simulink model "Hele_modellen_24_05_kl_20"  (R2022b)
settings: Solver=ode23t  StartTime=0.0  StopTime=3000  RelTol=1e-3
values from neighbouring files (symbols this model uses):
  A_stack_surface = 0.8*0.97*2+0.8*1.5*2+0.97*1.5*2    (= 6.862)    [Alle_konstanter_24_5_kl_20.m]
  c_p_stack = 870    [Alle_konstanter_24_5_kl_20.m]
  c_p_w = nyeretabelTcp.VarName2(1:250)    [Alle_konstanter_24_5_kl_20.m]
  cell_area = 5600    [Alle_konstanter_24_5_kl_20.m]
  ctc_an = 2    [Alle_konstanter_24_5_kl_20.m]
  ctc_ca = 2    [Alle_konstanter_24_5_kl_20.m]
  F = 96485.3321233100184    (= 96485.3321233)    [Alle_konstanter_24_5_kl_20.m]
  h_conv = 7.5    [Alle_konstanter_24_5_kl_20.m]
  i_0_an = 2*10^(-7)    (= 2e-07)    [Alle_konstanter_24_5_kl_20.m]
  i_0_ca = 2*10^(-3)    (= 0.002)    [Alle_konstanter_24_5_kl_20.m]
  idensdata = [0.746899 0.747476 0.748293 0.748876 0.749145 0.749908 0.750254 0.75072 0.751353 0.751779 0.752202 0.752682 ... (7200 elements, 90x80)]    [idensdata.mat]    (also in park_power.mat)
  lambda_m = 21    [Alle_konstanter_24_5_kl_20.m]
  M_H2 = 0.002016    [Alle_konstanter_24_5_kl_20.m]
  M_O2 = 0.031999    [Alle_konstanter_24_5_kl_20.m]
  m_stack = 2300    [Alle_konstanter_24_5_kl_20.m]
  N_cell = 36    [Alle_konstanter_24_5_kl_20.m]
  nr_of_stacks = 7    [Alle_konstanter_24_5_kl_20.m]
  P_lookup = 2:0.1:9.9    [Alle_konstanter_24_5_kl_20.m]
  R = 8.314    [Alle_konstanter_24_5_kl_20.m]
  T = transpose(1:250)    [Alle_konstanter_24_5_kl_20.m]
  T_amb = 20    [Alle_konstanter_24_5_kl_20.m]
  T_lookup = 283.15:1:372.15    [Alle_konstanter_24_5_kl_20.m]
  t_me = 175*10^(-4)    (= 0.0175)    [Alle_konstanter_24_5_kl_20.m]
  U_th = 1.473    [Alle_konstanter_24_5_kl_20.m]
undefined symbols (not defined in the file or in its folder): DiscIntNeverNeededParam
libraries: fl_lib x17, nesl_utility x10, ee_lib x2, SimscapeFluids_lib x1, simulink x1, dspsrcs4 x1
settings Model: Creator=drjon  LastModifiedBy=IrisM

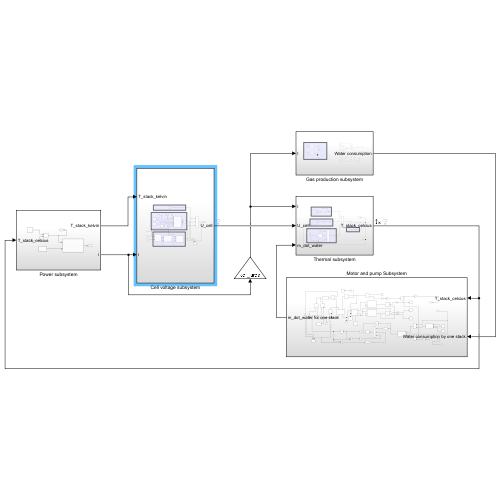
[thumbnail: Simulink's stored preview of the top-level diagram]
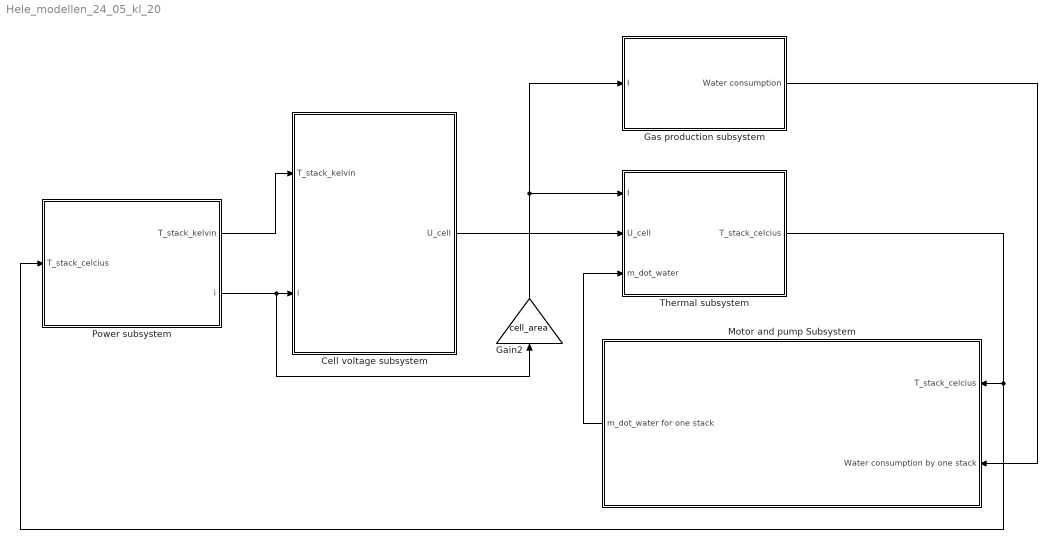
== system Hele_modellen_24_05_kl_20 ==
  Cell voltage subsystem : Subsystem
  Gain2 : Gain  Gain=cell_area
  Gas production subsystem : Subsystem
  Motor and pump Subsystem : Subsystem
  Power subsystem : Subsystem
  Thermal subsystem : Subsystem
  wires:
  Thermal subsystem/1(T_stack_celcius) -> Power subsystem/1(T_stack_celcius), Motor and pump Subsystem/1(T_stack_celcius)
  Cell voltage subsystem/1(U_cell) -> Thermal subsystem/2(U_cell)
  Gain2/1 -> Gas production subsystem/1(I), Thermal subsystem/1(I)
  Gas production subsystem/1(Water consumption) -> Motor and pump Subsystem/2(Water consumption by one stack)
  Motor and pump Subsystem/1(m_dot_water for one stack) -> Thermal subsystem/3(m_dot_water)
  Power subsystem/2(i) -> Cell voltage subsystem/2(i), Gain2/1
  Power subsystem/1(T_stack_kelvin) -> Cell voltage subsystem/1(T_stack_kelvin)

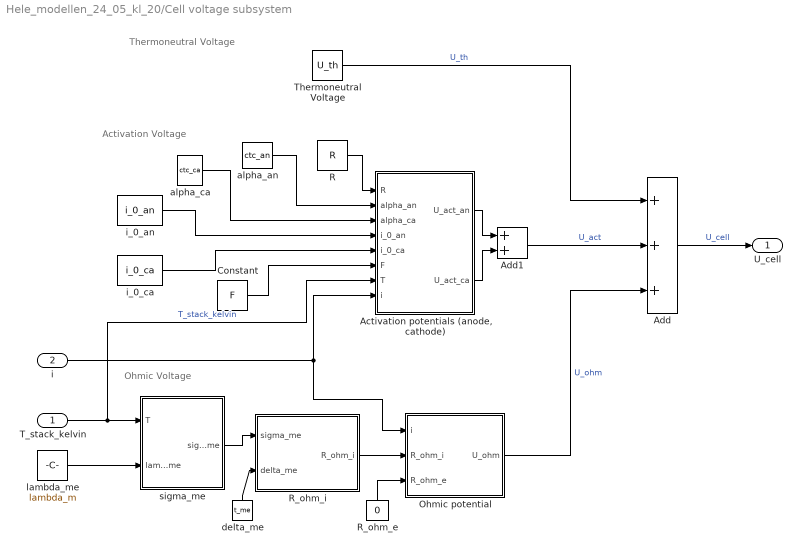
== system Hele_modellen_24_05_kl_20/Cell voltage subsystem ==
  note: Ohmic Voltage
  note: Activation Voltage
  note: Thermoneutral Voltage
  T_stack_kelvin : Inport
  i : Inport  Port=2
  "Activation potentials (anode, cathode)" : MATLAB Function  TreatAsAtomicUnit=on
  Add : Sum  Inputs=+++
  Add1 : Sum
  Constant : Constant  Value=F
  Ohmic potential : MATLAB Function  TreatAsAtomicUnit=on
  R : Constant  Value=R
  R_ohm_e : Constant  Value=0
  R_ohm_i : MATLAB Function  TreatAsAtomicUnit=on
  Thermoneutral Voltage : Constant  Value=U_th
  alpha_an : Constant  Value=ctc_an
  alpha_ca : Constant  Value=ctc_ca
  delta_me : Constant  Value=t_me
  i_0_an : Constant  Value=i_0_an
  i_0_ca : Constant  Value=i_0_ca
  lambda_me : Constant  Value=lambda_m
  sigma_me : MATLAB Function  TreatAsAtomicUnit=on
  U_cell : Outport
  wires:
  lambda_me/1 -> sigma_me/2(lambda_me)
  T_stack_kelvin/1 -> "Activation potentials (anode, cathode)"/7(T), sigma_me/1(T)  "T_stack_kelvin"
  i_0_an/1 -> "Activation potentials (anode, cathode)"/4(i_0_an)
  R/1 -> "Activation potentials (anode, cathode)"/1(R)
  i_0_ca/1 -> "Activation potentials (anode, cathode)"/5(i_0_ca)
  R_ohm_i/1(R_ohm_i) -> Ohmic potential/2(R_ohm_i)
  Add/1 -> U_cell/1  "U_cell"
  Add1/1 -> Add/2  "U_act"
  alpha_an/1 -> "Activation potentials (anode, cathode)"/2(alpha_an)
  delta_me/1 -> R_ohm_i/2(delta_me)
  Ohmic potential/1(U_ohm) -> Add/3  "U_ohm"
  sigma_me/1(sigma_me) -> R_ohm_i/1(sigma_me)
  alpha_ca/1 -> "Activation potentials (anode, cathode)"/3(alpha_ca)
  R_ohm_e/1 -> Ohmic potential/3(R_ohm_e)
  Constant/1 -> "Activation potentials (anode, cathode)"/6(F)
  Thermoneutral Voltage/1 -> Add/1  "U_th"
  "Activation potentials (anode, cathode)"/1(U_act_an) -> Add1/1
  "Activation potentials (anode, cathode)"/2(U_act_ca) -> Add1/2
  i/1 -> "Activation potentials (anode, cathode)"/8(i), Ohmic potential/1(i)

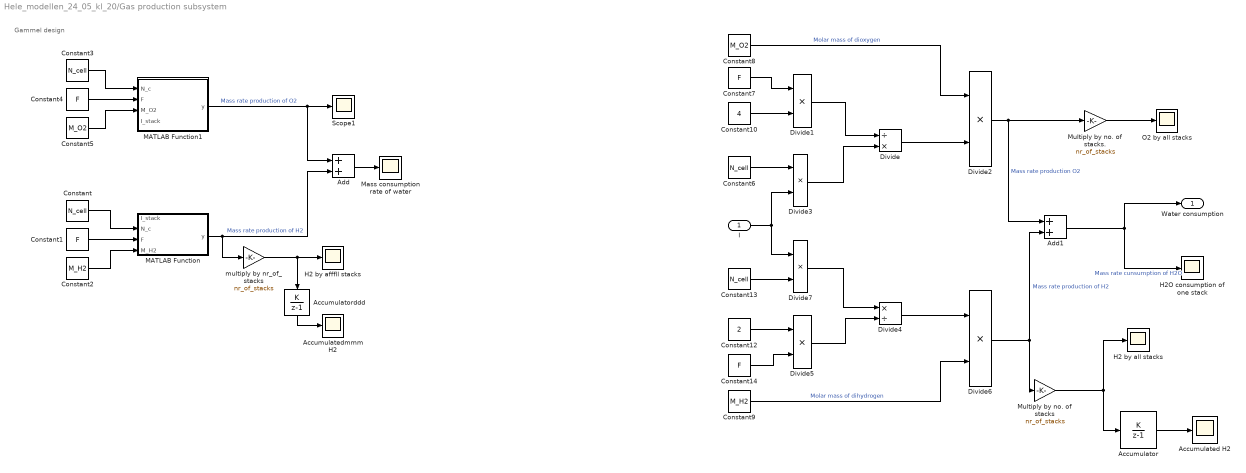
== system Hele_modellen_24_05_kl_20/Gas production subsystem ==
  note: Gammel design
  I : Inport
  Accumulated H2 : Scope
  Accumulatedmmm H2 : Scope
  Accumulator : DiscreteIntegrator  IntegratorMethod=Accumulation: Forward Euler  SampleTime=-1  ICPrevOutput=DiscIntNeverNeededParam  ICPrevScaledInput=DiscIntNeverNeededParam
  Accumulatorddd : DiscreteIntegrator  IntegratorMethod=Accumulation: Forward Euler  SampleTime=-1  ICPrevOutput=DiscIntNeverNeededParam  ICPrevScaledInput=DiscIntNeverNeededParam
  Add : Sum
  Add1 : Sum
  Constant{,3,6,13} (4 alike) : Constant  Value=N_cell
  Constant{1,4,7,14} (4 alike) : Constant  Value=F
  Constant10 : Constant  Value=4
  Constant12 : Constant  Value=2
  Constant2 : Constant  Value=M_H2
  Constant5 : Constant  Value=M_O2
  Constant8 : Constant  Value=M_O2
  Constant9 : Constant  Value=M_H2
  Divide : Product  Inputs=/*
  Divide{1..3,5..7} (6 alike) : Product  Inputs=**
  Divide4 : Product  Inputs=*/
  H2 by afffll stacks : Scope
  H2 by all stacks : Scope
  H2O consumption of one stack : Scope
  MATLAB Function : MATLAB Function  TreatAsAtomicUnit=on
  MATLAB Function1 : MATLAB Function  TreatAsAtomicUnit=on
  Mass consumption rate of water : Scope
  Multiply by no. of stacks : Gain  Gain=nr_of_stacks
  Multiply by no. of stacks. : Gain  Gain=nr_of_stacks
  O2 by all stacks : Scope
  Scope1 : Scope
  multiply by nr_of_stacks : Gain  Gain=nr_of_stacks
  Water consumption : Outport
  wires:
  MATLAB Function1/1(y) -> Add/1, Scope1/1  "Mass rate production of O2"
  Constant/1 -> MATLAB Function/2(N_c)
  Constant1/1 -> MATLAB Function/3(F)
  Add/1 -> Mass consumption rate of water/1
  Constant2/1 -> MATLAB Function/4(M_H2)
  Constant4/1 -> MATLAB Function1/2(F)
  MATLAB Function/1(y) -> Add/2, multiply by nr_of_stacks/1  "Mass rate production of H2"
  Constant5/1 -> MATLAB Function1/3(M_O2)
  Constant3/1 -> MATLAB Function1/1(N_c)
  multiply by nr_of_stacks/1 -> H2 by afffll stacks/1, Accumulatorddd/1
  Accumulatorddd/1 -> Accumulatedmmm H2/1
  Constant12/1 -> Divide5/1
  Constant7/1 -> Divide1/1
  Divide7/1 -> Divide4/1
  Divide3/1 -> Divide/2
  Multiply by no. of stacks/1 -> H2 by all stacks/1, Accumulator/1
  Divide4/1 -> Divide6/1
  Constant9/1 -> Divide6/2  "Molar mass of dihydrogen"
  Divide5/1 -> Divide4/2
  Constant14/1 -> Divide5/2
  Divide1/1 -> Divide/1
  Constant13/1 -> Divide7/2
  Constant8/1 -> Divide2/1  "Molar mass of dioxygen"
  Add1/1 -> Water consumption/1, H2O consumption of one stack/1  "Mass rate cunsumption of H2O"
  Constant10/1 -> Divide1/2
  Divide6/1 -> Add1/2, Multiply by no. of stacks/1  "Mass rate production of H2"
  Divide/1 -> Divide2/2
  Constant6/1 -> Divide3/1
  Divide2/1 -> Multiply by no. of stacks./1, Add1/1  "Mass rate production O2"
  Accumulator/1 -> Accumulated H2/1
  I/1 -> Divide7/1, Divide3/2
  Multiply by no. of stacks./1 -> O2 by all stacks/1

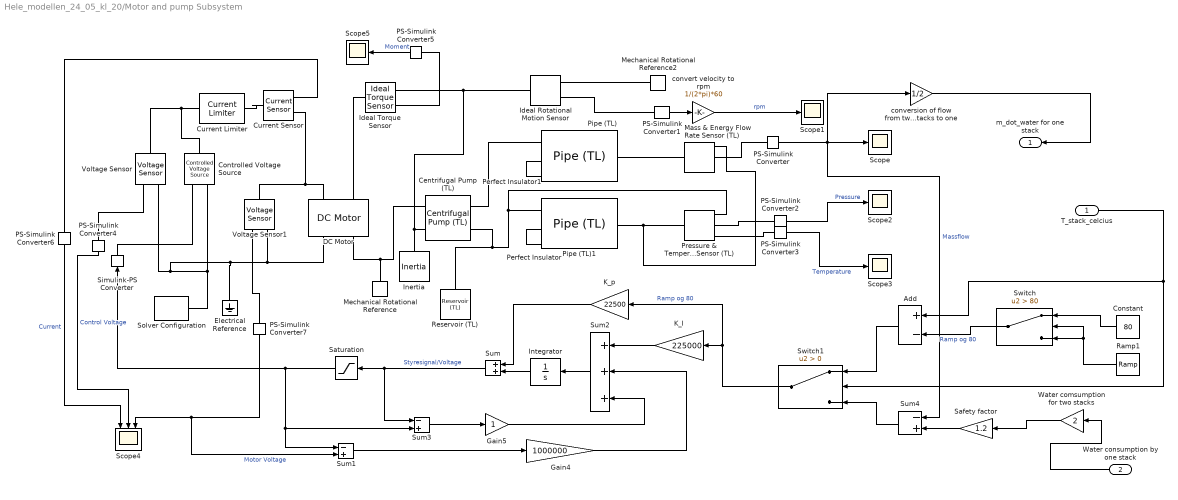
== system Hele_modellen_24_05_kl_20/Motor and pump Subsystem ==
  T_stack_celcius : Inport
  Water consumption by one stack : Inport  Port=2
  Add : Sum  Inputs=+-
  Centrifugal Pump (TL) : SimscapeFluids_lib/Thermal Liquid/Pumps & Motors/Centrifugal Pump (TL)  pump_parameterization=fluids.thermal_liquid.pumps_motors.enum.CentrifugalPumpParameterization.Nominal  capacity_ref_nominal=290 lpm  head_ref_nominal=40 m  power_ref_nominal=0.85 kW  head_ref_max=60 m  capacity_ref_max=300 lpm  omega_ref_analytic=1150 rpm  flow_rate_1D_TLU=[16.67, 30, 40, 53.33, 66.67, 83.33] lpm  head_1D_TLU=[50, 47.5, 45, 40, 35, 25] m  power_1D_TLU=[.6, .75, .85, .93, .98, .99] kW  omega_ref_1D=3500 rpm  rho_ref_1D=998.21 kg/m^3  flow_rate_2D_TLU=[16.67, 23.33, 30, 40, 53.33, 60] lpm  omega_2D_TLU=[2450, 2800, 3150, 3500] rpm  head_2D_TLU=[25, 32.7, 42.5, 50; 24, 31.7, 41, 49; 22.7, 30.5, 39, 47.5; 20, 28, 36, 45; 15.7, 24, 32, 40; 12.5, 21, 29.5, 37.5] m  power_2D_TLU=[.28, .38, .5, .6; .31, .41, .55, .68; .33, .44, .6, .75; .36, .48, .65, .83; .38, .53, .72, .93; .39, .55, .75, .97] kW  rho_ref_2D=998.21 kg/m^3  diameter_ratio=1  mech_orientation=fluids.thermal_liquid.pumps_motors.enum.CentrifugalPumpMechOrientation.Positive  area=0.01 m^2
      settings: InternalSimscapePortConfiguration="{\"Bottom\":[],\"Left\":[{\"id\":\"A\",\"label\":\"A\",\"type\":\"foundation.thermal_liquid.thermal_liquid\"},{\"id\":\"B\",\"label\":\"B\",\"type\":\"foundation.thermal_liquid.thermal_liquid\"}],\"Right\":[{\"id\":\"R\",\"label\":\"R\",\"type\":\"foundation.mechanical.rotational.rotational\"},{\"id\":\"C\",\"label\":\"C\",\"type\":\"foundation.mechanical.rotational.rotational\"}],\"Top\":[]}"
  Constant : Constant  Value=80
  Controlled Voltage Source : fl_lib/Electrical/Electrical Sources/Controlled Voltage Source
  Current Limiter : ee_lib/Semiconductors & Converters/Current Limiter  iLim=4.5 A  vLim=0.1 V  gLim=1e-9 1/Ohm  thermal_mass=100 J/K  initial_temperature=298.15 K
      settings: InternalSimscapePortConfiguration="{\"Bottom\":[],\"Left\":[{\"id\":\"p\",\"label\":\"+\",\"type\":\"foundation.electrical.electrical\"}],\"Right\":[{\"id\":\"n\",\"label\":\"-\",\"type\":\"foundation.electrical.electrical\"}],\"Top\":[]}"
  Current Sensor : fl_lib/Electrical/Electrical Sensors/Current Sensor
  DC Motor : ee_lib/Electromechanical/Brushed Motors/DC Motor  field_option=ee.enum.field_option.pm  Rf=100 Ohm  Lf=1 H  Laf=0.15 H  If0=0 A  parameterization=ee.enum.dcparam_option.circuit_param  Ra=3.9 Ohm  La=14e-3 H  emf_or_torque=ee.enum.emf_or_torque.kv  Kv=1.2 V/(rad/s)  Ki=6.876e-4 N*m/A  T_stall=0.24e-3 N*m  w_max=19100 rpm  w_rated=15000 rpm  P_rated=0.08 W  V_rated=1.5 V  lam_param=ee.enum.lam_param.damping  i_noload=0 A  V_i_noload=1.5 V  J=0.00088 kg*m^2  lam=0 N*m*s/rad  speed0=0 rpm  enable_fault_armature=simscape.enum.onoff.off  rev_faulted=1 / 3  G_faulted_armature=1e-5 S  fault_trigger_armature=ee.enum.faults.faultTrigger.temporal  t_fault_armature=1 s  max_permissible_current_armature=inf A  t_fail_on_current_armature=1 s  enable_fault_field=simscape.enum.onoff.off  G_faulted_field=1e-5 S  fault_trigger_field=ee.enum.faults.faultTrigger.temporal  t_fault_field=1 s  max_permissible_current_field=inf A  t_fail_on_current_field=1 s  fault_action=simscape.enum.assert.action.none  alpha=3.93e-3 1/K  Tmeas=25 degC  thermal_mass=100 J/K  initial_temperature=25 degC
  Electrical Reference : fl_lib/Electrical/Electrical Elements/Electrical Reference
  Gain4 : Gain  Gain=1000000
  Gain5 : Gain
  Ideal Rotational Motion Sensor : fl_lib/Mechanical/Mechanical Sensors/Ideal Rotational Motion Sensor  reference=foundation.enum.MeasurementReference.difference  acceleration_port=false  velocity_port=true  position_port=false  wrap_angle=false  offset=0 rad
      settings: InternalSimscapePortConfiguration="{\"Bottom\":[],\"Left\":[{\"id\":\"R\",\"label\":\"R\",\"type\":\"foundation.mechanical.rotational.rotational\"}],\"Right\":[{\"id\":\"C\",\"label\":\"C\",\"type\":\"foundation.mechanical.rotational.rotational\"},{\"id\":\"W\",\"label\":\"W\",\"type\":\"output\"}],\"Top\":[]}"
  Ideal Torque Sensor : fl_lib/Mechanical/Mechanical Sensors/Ideal Torque Sensor
  Inertia : fl_lib/Mechanical/Rotational Elements/Inertia  inertia=0.000176 kg*m^2  num_ports=foundation.enum.numPorts2.one  w_specify=off  w_priority=High  w=0 rad/s  w_nominal_specify=off  w_nominal_unit=rad/s  w_nominal_value=1  t_specify=off  t_priority=None  t=0 N*m  t_nominal_specify=off  t_nominal_unit=N*m  t_nominal_value=1
  Integrator : Integrator
  K_I : Gain  Gain=225000
  K_p : Gain  Gain=22500
  Mass & Energy Flow Rate Sensor (TL) : fl_lib/Thermal Liquid/Sensors/Mass & Energy Flow Rate Sensor (TL)
      settings: InternalSimscapePortConfiguration="{\"Bottom\":[],\"Left\":[{\"id\":\"A\",\"label\":\"A\",\"type\":\"foundation.thermal_liquid.thermal_liquid\"}],\"Right\":[{\"id\":\"B\",\"label\":\"B\",\"type\":\"foundation.thermal_liquid.thermal_liquid\"},{\"id\":\"M\",\"label\":\"M\",\"type\":\"output\"},{\"id\":\"PHI\",\"label\":\"Phi\",\"type\":\"output\"}],\"Top\":[]}"
  Mechanical Rotational Reference : fl_lib/Mechanical/Rotational Elements/Mechanical Rotational Reference
  Mechanical Rotational Reference2 : fl_lib/Mechanical/Rotational Elements/Mechanical Rotational Reference
  PS-Simulink Converter{,1..7} (8 alike) : nesl_utility/PS-Simulink Converter  PhysicalDomain=network_engine_domain  SubClassName=ps_output  LeftPortType=input  RightPortType=output  PseudoPeriodic=off  Frequencies=[]  VectorFormat=inherit  Unit=inherit  AffineConversion=off
  Perfect Insulator : fl_lib/Thermal/Thermal Elements/Perfect Insulator  T_specify=off  T_priority=None  T=293.15 K  T_nominal_specify=off  T_nominal_unit=K  T_nominal_value=1
  Perfect Insulator1 : fl_lib/Thermal/Thermal Elements/Perfect Insulator  T_specify=off  T_priority=None  T=293.15 K  T_nominal_specify=off  T_nominal_unit=K  T_nominal_value=1
  Pipe (TL) : fl_lib/Thermal Liquid/Elements/Pipe (TL)  length=5 m  area=0.01 m^2  Dh=0.1128 m  length_add=1 m  roughness=15e-6 m  Re_lam=2000  Re_tur=4000  shape_factor=64  Nu_lam=3.66  dynamic_compressibility=simscape.enum.onoff.on  inertia=simscape.enum.onoff.off  p0=3.5 MPa  T0=293.15 K  mdot0=0 kg/s
  Pipe (TL)1 : fl_lib/Thermal Liquid/Elements/Pipe (TL)  length=5 m  area=0.01 m^2  Dh=0.1128 m  length_add=1 m  roughness=15e-6 m  Re_lam=2000  Re_tur=4000  shape_factor=64  Nu_lam=3.66  dynamic_compressibility=simscape.enum.onoff.on  inertia=simscape.enum.onoff.off  p0=3.5 MPa  T0=293.15 K  mdot0=0 kg/s
  Pressure & Temperature Sensor (TL) : fl_lib/Thermal Liquid/Sensors/Pressure & Temperature Sensor (TL)
      settings: InternalSimscapePortConfiguration="{\"Bottom\":[],\"Left\":[{\"id\":\"A\",\"label\":\"A\",\"type\":\"foundation.thermal_liquid.thermal_liquid\"}],\"Right\":[{\"id\":\"B\",\"label\":\"B\",\"type\":\"foundation.thermal_liquid.thermal_liquid\"},{\"id\":\"P\",\"label\":\"P\",\"type\":\"output\"},{\"id\":\"T\",\"label\":\"T\",\"type\":\"output\"}],\"Top\":[]}"
  Ramp1 : simulink/Sources/Ramp  slope=0.05  start=0  InitialOutput=20
  Reservoir (TL) : fl_lib/Thermal Liquid/Elements/Reservoir (TL)  pressure_spec=foundation.enum.pressure_spec.specified  reservoir_pressure=3.5 MPa  reservoir_temperature=293.15 K  area=0.01 m^2
  Safety factor : Gain  Gain=1.2
  Saturation : Saturate  UpperLimit=300  LowerLimit=0
  Scope{,1..3,5} (5 alike) : Scope
  Scope4 : Scope  NumInputPorts=3
  Simulink-PS Converter : nesl_utility/Simulink-PS Converter  PhysicalDomain=network_engine_domain  SubClassName=ps_input  LeftPortType=input  RightPortType=output  PseudoPeriodic=off  Frequencies=[]  NoiseDistribution=none  NoiseParameters=[]  Unit=1  AffineConversion=off  FilteringAndDerivatives=provide  SimscapeFilterOrder=1  InputFilterTimeConstant=0.001  UdotUserProvided=0
  Solver Configuration : nesl_utility/Solver Configuration  PhysicalDomain=network_engine_domain  SubClassName=solver  LeftPortType=input  RightPortType=generic  Tones=[]  Harmonics=[]  SimulateNoise=off  Profile=off  UseLocalSampling=off  EnableSwitchedLinearOptims=on  FrequencyDomain=off  UseCCode=off  RelTol=0.001  AbsTol=0.001  MinStep=1e-09  ToWorkspace=off  RevertToSquareIcSolve=off  NumHomotopyIterations=100  PhasorMode=off  PhasorModeNumHarmonics=1  ConsistencySolver=NEWTON_XTOL_AFTER_FTOL  IndexReductionMethod=DerivativeReplacement  DoDC=off  ResidualTolerance=1e-09  ConsistencyTolSource=GLOBAL  ConsistencyAbsTol=0.001  ConsistencyRelTol=0.001  ConsistencyTolFactor=0.001  UseLocalSolver=off  LocalSolverChoice=NE_BACKWARD_EULER_ADVANCER  ResolveIndetEquations=on  FunctionEvalNumThread=1  LocalSolverSampleTime=0.001  DoFixedCost=off  MaxNonlinIter=3  MaxModeIter=2  ComputeImpulses=off  ImpulseIterations=2  LinearAlgebra=auto  LinearAlgebraNumThread=0  EquationFormulation=NE_TIME_EF  DelaysMemoryBudget=1024  AutomaticFiltering=on  FilteringTimeConstant=0.001  PartitionStorageMethod=AS_NEEDED  PartitionMemoryBudget=1024  PartitionMethod=ROBUST
  Sum : Sum
  Sum1 : Sum  Inputs=-+
  Sum2 : Sum  Inputs=+++
  Sum3 : Sum  Inputs=-+
  Sum4 : Sum  Inputs=-+
  Switch : Switch  Criteria=u2 > Threshold  Threshold=80  SaturateOnIntegerOverflow=off  InputSameDT=off
  Switch1 : Switch  Criteria=u2 > Threshold  SaturateOnIntegerOverflow=off  InputSameDT=off
  Voltage Sensor : fl_lib/Electrical/Electrical Sensors/Voltage Sensor
  Voltage Sensor1 : fl_lib/Electrical/Electrical Sensors/Voltage Sensor
  Water comsumption for two stacks : Gain  Gain=2
  conversion of flow from two stacks to one : Gain  Gain=1/2
  convert velocity to rpm : Gain  Gain=1/(2*pi)*60
  m_dot_water for one stack : Outport
  wires:
  PS-Simulink Converter/1 -> Scope/1, Sum4/1, conversion of flow from two stacks to one/1  "Massflow"
  PS-Simulink Converter3/1 -> Scope3/1  "Temperature"
  PS-Simulink Converter6/1 -> Scope4/1  "Current"
  Switch1/1 -> K_p/1, K_I/1  "Ramp og 80"
  Saturation/1 -> Sum1/1, Sum3/2, Simulink-PS Converter/1
  T_stack_celcius/1 -> Switch1/2, Add/1
  Water consumption by one stack/1 -> Water comsumption for two stacks/1
  PS-Simulink Converter2/1 -> Scope2/1  "Pressure"
  PS-Simulink Converter1/1 -> convert velocity to rpm/1
  Sum/1 -> Sum3/1, Saturation/1  "Styresignal/Voltage"
  Ramp1/1 -> Switch/2, Switch/3
  PS-Simulink Converter5/1 -> Scope5/1  "Moment"
  Add/1 -> Switch1/1
  PS-Simulink Converter4/1 -> Scope4/2  "Control Voltage"
  Sum2/1 -> Integrator/1
  K_I/1 -> Sum2/1
  Constant/1 -> Switch/1
  convert velocity to rpm/1 -> Scope1/1  "rpm"
  PS-Simulink Converter7/1 -> Sum1/2, Scope4/3  "Motor Voltage"
  Gain5/1 -> Sum2/3
  Sum3/1 -> Gain5/1
  Integrator/1 -> Sum/2
  Gain4/1 -> Sum2/2
  Sum1/1 -> Gain4/1
  Water comsumption for two stacks/1 -> Safety factor/1
  Safety factor/1 -> Sum4/2
  K_p/1 -> Sum/1
  Switch/1 -> Add/2  "Ramp og 80"
  conversion of flow from two stacks to one/1 -> m_dot_water for one stack/1
  Sum4/1 -> Switch1/3
  connections:
  Inertia/LConn1 -- Ideal Rotational Motion Sensor/LConn1 -- Ideal Torque Sensor/RConn1 -- Centrifugal Pump (TL)/RConn1
  Mechanical Rotational Reference2/LConn1 -- Ideal Rotational Motion Sensor/RConn1
  PS-Simulink Converter3/LConn1 -- Pressure & Temperature Sensor (TL)/RConn3
  Ideal Torque Sensor/LConn1 -- DC Motor/LConn2
  Ideal Rotational Motion Sensor/RConn2 -- PS-Simulink Converter1/LConn1
  Mass & Energy Flow Rate Sensor (TL)/RConn1 -- Pressure & Temperature Sensor (TL)/LConn1 -- Pipe (TL)1/RConn1
  Mechanical Rotational Reference/LConn1 -- Centrifugal Pump (TL)/RConn2 -- DC Motor/RConn2
  Current Limiter/LConn1 -- Voltage Sensor/LConn1 -- Controlled Voltage Source/LConn1
  PS-Simulink Converter2/LConn1 -- Pressure & Temperature Sensor (TL)/RConn2
  Centrifugal Pump (TL)/LConn2 -- Pipe (TL)/LConn1
  PS-Simulink Converter/LConn1 -- Mass & Energy Flow Rate Sensor (TL)/RConn2
  Pipe (TL)1/LConn1 -- Centrifugal Pump (TL)/LConn1 -- Reservoir (TL)/LConn1 -- Pressure & Temperature Sensor (TL)/RConn1
  DC Motor/LConn1 -- Current Sensor/RConn2 -- Voltage Sensor1/LConn1
  Current Sensor/LConn1 -- Current Limiter/RConn1
  DC Motor/RConn1 -- Electrical Reference/LConn1 -- Controlled Voltage Source/RConn2 -- Solver Configuration/RConn1 -- Voltage Sensor/RConn2 -- Voltage Sensor1/RConn2
  Perfect Insulator/LConn1 -- Pipe (TL)1/LConn2
  Voltage Sensor1/RConn1 -- PS-Simulink Converter7/LConn1
  Mass & Energy Flow Rate Sensor (TL)/LConn1 -- Pipe (TL)/RConn1
  Controlled Voltage Source/RConn1 -- Simulink-PS Converter/RConn1
  Ideal Torque Sensor/RConn2 -- PS-Simulink Converter5/LConn1
  PS-Simulink Converter4/LConn1 -- Voltage Sensor/RConn1
  Perfect Insulator1/LConn1 -- Pipe (TL)/LConn2
  Current Sensor/RConn1 -- PS-Simulink Converter6/LConn1

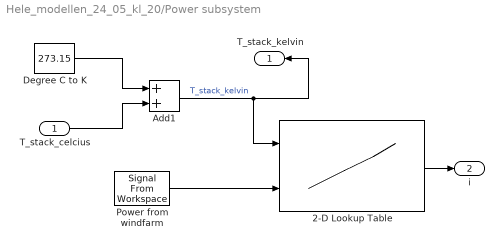
== system Hele_modellen_24_05_kl_20/Power subsystem ==
  T_stack_celcius : Inport
  2-D Lookup Table : Lookup_n-D  BreakpointsForDimension1=T_lookup  BreakpointsForDimension2=P_lookup  Table=idensdata  InternalRulePriority=Speed  RndMeth=Simplest
      settings: InputPortMap=u0,u1
  Add1 : Sum
  Degree C to K : Constant  Value=273.15
  Power from windfarm : dspsrcs4/Signal From Workspace  X=park_power  Ts=1  nsamps=1  OutputAfterFinalValue=Setting to zero  ignoreOrWarnInputAndFrameLengths=off  OutputFrames=off
  T_stack_kelvin : Outport
  i : Outport  Port=2
  wires:
  Add1/1 -> 2-D Lookup Table/1, T_stack_kelvin/1  "T_stack_kelvin"
  Degree C to K/1 -> Add1/1
  T_stack_celcius/1 -> Add1/2
  Power from windfarm/1 -> 2-D Lookup Table/2
  2-D Lookup Table/1 -> i/1

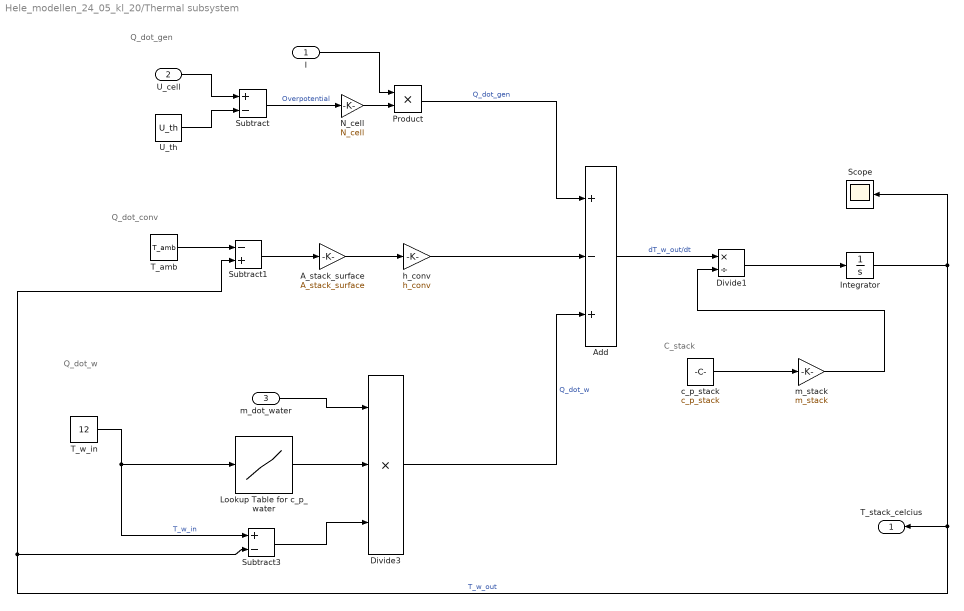
== system Hele_modellen_24_05_kl_20/Thermal subsystem ==
  note: C_stack
  note: Q_dot_w
  note: Q_dot_conv
  note: Q_dot_gen
  I : Inport
  U_cell : Inport  Port=2
  m_dot_water : Inport  Port=3
  A_stack_surface : Gain  Gain=A_stack_surface
  Add : Sum  Inputs=+-+
  Divide1 : Product  Inputs=*/
  Divide3 : Product  Inputs=***
  Integrator : Integrator  InitialCondition=T_amb
  Lookup Table for c_p_water : Lookup_n-D  NumberOfTableDimensions=1  BreakpointsForDimension1=T  Table=c_p_w  InternalRulePriority=Speed  RndMeth=Simplest
  N_cell : Gain  Gain=N_cell
  Product : Product
  Scope : Scope
  Subtract : Sum  Inputs=+-
  Subtract1 : Sum  Inputs=-+
  Subtract3 : Sum  Inputs=+-
  T_amb : Constant  Value=T_amb
  T_w_in : Constant  Value=12
  U_th : Constant  Value=U_th
  c_p_stack : Constant  Value=c_p_stack
  h_conv : Gain  Gain=h_conv
  m_stack : Gain  Gain=m_stack
  T_stack_celcius : Outport
  wires:
  U_th/1 -> Subtract/2
  Lookup Table for c_p_water/1 -> Divide3/2
  T_w_in/1 -> Subtract3/1, Lookup Table for c_p_water/1  "T_w_in"
  Product/1 -> Add/1  "Q_dot_gen"
  h_conv/1 -> Add/2
  Subtract/1 -> N_cell/1  "Overpotential"
  Divide3/1 -> Add/3  "Q_dot_w"
  N_cell/1 -> Product/2
  Integrator/1 -> Subtract1/2, Subtract3/2, T_stack_celcius/1, Scope/1  "T_w_out"
  T_amb/1 -> Subtract1/1
  Subtract1/1 -> A_stack_surface/1
  A_stack_surface/1 -> h_conv/1
  Subtract3/1 -> Divide3/3
  c_p_stack/1 -> m_stack/1
  I/1 -> Product/1
  U_cell/1 -> Subtract/1
  m_dot_water/1 -> Divide3/1
  Add/1 -> Divide1/1  "dT_w_out/dt"
  m_stack/1 -> Divide1/2
  Divide1/1 -> Integrator/1

== matlab function Hele_modellen_24_05_kl_20/Cell voltage subsystem/sigma_me ==
  data: T input; lambda_me input; sigma_me output
function sigma_me = f(T, lambda_me)
sigma_me = (0.00514*lambda_me - 0.00326)*exp(1268*(1/303-1/T));

f = sigma_me;

== matlab function Hele_modellen_24_05_kl_20/Cell voltage subsystem/Ohmic potential ==
  data: i input; R_ohm_i input; R_ohm_e input; U_ohm output
%% Ohmic overpotential calculations

function U_ohm = f(i, R_ohm_i,R_ohm_e)
U_ohm = i*(R_ohm_i+R_ohm_e); 

f = U_ohm;

== matlab function Hele_modellen_24_05_kl_20/Cell voltage subsystem/Activation potentials (anode, cathode) ==
  data: R input; alpha_an input; alpha_ca input; i_0_an input; i_0_ca input; F input; T input; i input; U_act_an output; U_act_ca output
function [U_act_an, U_act_ca] = f(R, alpha_an, alpha_ca, i_0_an, i_0_ca, F, T, i)
U_act_an =(R*T/(F*alpha_an))*asinh(i/(2*i_0_an));
U_act_ca = (R*T/(F*alpha_ca))*asinh(i/(2*i_0_ca));

f = U_act_ca;
f = U_act_an ;

== matlab function Hele_modellen_24_05_kl_20/Cell voltage subsystem/R_ohm_i ==
  data: sigma_me input; R_ohm_i output; delta_me input
function R_ohm_i = f(sigma_me, delta_me)
R_ohm_i = delta_me/sigma_me; 

f = R_ohm_i;

== matlab function Hele_modellen_24_05_kl_20/Gas production subsystem/MATLAB Function ==
  data: I_stack input; y output; N_c input; F input; M_H2 input
function y = fcn(I_stack,N_c,F,M_H2) % Operation current [A]

N_dot_H2_g=N_c*I_stack/(2*F); %mol H2/sekund

m_dot_H2_g=N_dot_H2_g*M_H2; %Kg H2/sekund

y=m_dot_H2_g;

== matlab function Hele_modellen_24_05_kl_20/Gas production subsystem/MATLAB Function1 ==
  data: N_c input; F input; M_O2 input; I_stack input; y output
function y = fcn(N_c,F,M_O2,I_stack) % Operation current [A]

N_dot_O2_g=N_c*I_stack/(4*F); %mol O2/sekund

m_dot_O2_g=N_dot_O2_g*M_O2; %Kg O2/sekund

y=m_dot_O2_g;
